simulink library "library_BCM"  (Simulink 8.2)
settings: Solver=ode45  StartTime=0.0  StopTime=10.0  RelTol=1e-3
undefined symbols (not defined in the file or in its folder): MPU_FOUR_CST, MPU_ONE_CST, MPU_THREE_CST, MPU_TWO_CST, MPU_ZERO_CST, NAMEOFTHEMODEL_SAMPLE_TIME_CST, slcm, TYP_MPU_REQUEST, TYP_MPU_REQUEST_2, TYP_MPU_STATUS, TYP_MPU_STATUS_2
libraries: Renault_Library x50, simulink x8, library_BCM x7
(part 1 of 3)
Description:
  | Library_BCM v1.0 :
  | Creation
  | Library_BCM v1.2 :
  | Corrections in Fault Manager
  | Library_BCM v1.3 :
  | Add MPU example in Modeling
  | Library_BCM v1.4 :
  | Add Block Conv_BoolToEvent_RisingEdge in Modeling
  | Library_BCM v1.5 :
  | Corrections in Fault Manager
  | Library_BCM v1.6 :
  | Add block EEPROM_SIMU in Validation
  | Library_BCM v.1.7 :
  | Add block EEPROM RNTBCI in Validation
  | Library_BCM v.1.8 :
  | Corrections of block EEPROM_SNAPSHOT in Fault Manager
  | Library_BCM v.1.9 :
  | Corrections of block EEPROM_SNAPSHOT in Fault Manager
  | Library_BCM v.1.10 :
  | Corrections of block CAN_FRAME_PRESENCE
  | Library_BCM v.1.11 :
  | Corrections of block EEPROM_SNAPSHOT in Fault Manager
  | Library_BCM v.1.12 :
  | Add  block PRESOAK_CHARGE_5CAL_7DAY
  | Library_BCM v.1.13 :
  | Optimisation of blocks in Fault Manager
  | Library_BCM v.1.14 :
  | correction of block EEPROM in Fault Manager
  | Library_BCM v.1.15 :
  | correction of block EEPROM in Fault Manager
  | Library_BCM v.1.16 :
  | correction of block EEPROM in Fault Manager
  | Library_BCM v.1.17 :
  | correction of block DTC & EEPROM in Fault Manager
  | Library_BCM v.1.18 :
  | correction of block EEPROM in Fault Manager
  | Library_BCM v.1.19 :
  | correction of block EEPROM in Fault Manager
  | Library_BCM v.1.20 :
  | correction of block DTC in Fault Manager
  | Library_BCM v.1.21 :
  | correction of block DTC in Fault Manager
  | Library_BCM v.1.22 :
  | correction of block INITIAL_PARAMETER in MIL Full Matlab
  | Library_BCM v.1.23 :
  | correction of block EEPROM in Fault Manager (RESET/RAZ)
  | Library_BCM v.1.24 :
  | add block RSA_Dynamic2DLockupTable : ver : 01.00 for clim waiting included in library lite
  | Library_BCM v.1.25 :
  | correction of block EEPROM in Fault Manager (constant type, QA FNR)
  | Library_BCM v.1.26 :
  | Correction of block RSA_Dynamic2DLockupTable to delete double inside
settings Model: Creator=p072376  LastModifiedBy=a003809

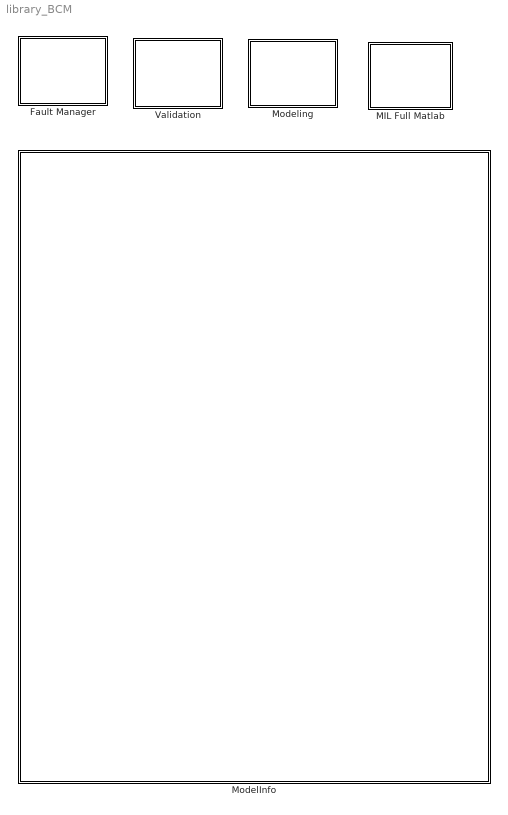
== system library_BCM ==
  Fault Manager : Subsystem
  MIL Full Matlab : Subsystem
  ModelInfo : Subsystem  LoadFcn=slcm LoadBlock;  InitFcn=slcm('UpdateAllCMBlocksInThisModelInit')  mask(CMBlock){InitialSaveTempField=, InitialBlockCM=None, BlockCM=None, Frame=on, SaveTempField=, DisplayStringWithTags=|, MaskDisplayString=library_BCM\nLibrary_BCM v1.0 : \nCreation\nLibrary_BCM v1.2 :\nCorrections in Fault Manager\nLibrary_BCM v1.3 :\nAdd MPU example in Modeling\nLibrary_BCM v1.4 :\nAdd Block Conv_BoolToEvent_RisingEdge in Modeling\nLibrary_BCM v1.5 :\nCorrections in Fault Manager\nLibrary_BCM v1.6 :\nAdd block EEPROM_SIMU in Validation\nLibrary_BCM v.1.7 :\nAdd block EEPROM RNTBCI in Validation\nLibrary_BCM v.1.8 :\nCorrections of block EEPROM_SNAPSHOT in Fault Manager\nLibrary_BCM v.1.9 :\nCorrections of block EEPROM_SNAPSHOT in Fault Manager\nLibrary_BCM v.1.10 :\nCorrections of block CAN_FRAME_PRESENCE\nLibrary_BCM v.1.11 :\nCorrections of block EEPROM_SNAPSHOT in Fault Manager\nLibrary_BCM v.1.12 :\nAdd  block PRESOAK_CHARGE_5CAL_7DAY\nLibrary_BCM v.1.13 :\nOptimisation of blocks in Fault Manager\nLibrary_BCM v.1.14 :\ncorrection of block EEPROM in Fault Manager\nLibrary_BCM v.1.15 :\ncorrection of block EEPROM in Fault Manager\nLibrary_BCM v.1.16 :\ncorrection of block EEPROM in Fault Manager\nLibrary_BCM v.1.17 :\ncorrection of block DTC & EEPROM in Fault Manager\nLibrary_BCM v.1.18 :\ncorrection of block EEPROM in Fault Manager\nLibrary_BCM v.1.19 :\ncorrection of block EEPROM in Fault Manager\nLibrary_BCM v.1.20 :\ncorrection of block DTC in Fault Manager\nLibrary_BCM v.1.21 :\ncorrection of block DTC in Fault Manager\nLibrary_BCM v.1.22 :\ncorrection of block INITIAL_PARAMETER in MIL Full Matlab\nLibrary_BCM v.1.23 :\ncorrection of block EEPROM in Fault Manager (RESET/RAZ)\nLibrary_BCM v.1.24 :\nadd block RSA_Dynamic2DLockupTable : ver : 01.00 for clim waiting included in library lite\nLibrary_BCM v.1.25 :\ncorrection of block EEPROM in Fault Manager (constant type, QA FNR)\nLibrary_BCM v.1.26 :\nCorrection of block RSA_Dynamic2DLockupTable to delete double inside, HorizontalTextAlignment=Center, LeftAlignmentValue=0.5, SourceBlockDiagram=library_BCM, TagMaxNumber=20, CMTag1=, CMTag2=, CMTag3=, CMTag4=, CMTag5=, CMTag6=, CMTag7=, CMTag8=, CMTag9=, CMTag10=, CMTag11=, CMTag12=, CMTag13=, CMTag14=, CMTag15=, CMTag16=, CMTag17=, CMTag18=, CMTag19=, CMTag20=}
      mask DisplayStringWithTags=|
      | %<ModelName>
      | %<Description>
      mask help: This block allows revision control information to be displayed within the model.
      settings: CopyFcn=slcm CopyBlock;  DeleteFcn=slcm Cancel;  PostSaveFcn=slcm('UpdateAllCMBlocksInThisModel')  NameChangeFcn=slcm Rename;  OpenFcn=slcm
      mask Display: text(str2num(LeftAlignmentValue), 0.5, MaskDisplayString, 'HorizontalAlignment', HorizontalTextAlignment)
  Modeling : Subsystem
  Validation : Subsystem

== system library_BCM/Fault Manager ==
  DTC : Subsystem  Tag=[RUNNABLE]  Description=|  mask{DTC_IDENTITY=928514, DTC_SNAPSHOT_NUMBER_CONV_CST=3, NUMBER_DTC_RECORD_IN_E2P_CST=2}
      | RQT_Fault_Manager_BCM_1_1
      | RQT_Fault_Manager_BCM_1_2
      | RQT_Fault_Manager_BCM_2_1
      | RQT_Fault_Manager_BCM_2_5
      mask prompts: DTC_IDENTITY "identification number DTC"; DTC_SNAPSHOT_NUMBER_CONV_CST "snapshot number"; NUMBER_DTC_RECORD_IN_E2P_CST "Number of DTC save in EEPROM"
  EEPROM_SNAPSHOT : Subsystem  mask{NUMBER_DTC_RECORD_IN_RAM_CST=178, NUMBER_DTC_RECORD_IN_E2P_CST=10, SNAPSHOT_NUMBER_CST=5, SNAPSHOT_MAX_LENGHT=32}
      mask prompts: NUMBER_DTC_RECORD_IN_RAM_CST "Number of DTC"; NUMBER_DTC_RECORD_IN_E2P_CST "Number of DTC save in EEPROM"; SNAPSHOT_NUMBER_CST "Number of snapshot"; SNAPSHOT_MAX_LENGHT "Snapshot max lenght (octet)"

== system library_BCM/MIL Full Matlab ==
  CAN_FRAME_PRESENCE : Subsystem  Tag=[REUSABLE]
  CONVERT_INT_TO_ENUM_WITH_UNAVAILABLE_VALUE : Subsystem  mask{UnavailableValue=3}
      mask prompts: UnavailableValue "Unavailable Value"
  COUNTER_INC : Subsystem
  INITIAL_PARAMETER : Subsystem  mask{INITIAL_VALUE=[9 99 100]}
  MONITORED_FRAME_MANAGEMENT : Subsystem  mask{CycleTime=10}
      mask prompts: CycleTime "Cycle Time in Ms"
  MUX_SEND_FRAME : Subsystem  mask(RSA_MuxSendFrame){FRAME_PERIOD=10, MAX_PARAMETER=3}
      mask prompts: FRAME_PERIOD "Period (ms)"; MAX_PARAMETER "Max counter"
      mask help:
      | Send a frame periodically or when an event parameter is updated.
      | - Period: Frame period (in ms)
      | Version : 01.00
      mask Help:
      | Send a frame periodically or when an event parameter is updated.
      | - Period: Frame period (in ms)
      | Version : 01.00
      mask Display:
      | disp('Mux Send Frame Simulink')
      | port_label('Input',1,'CAN_V_EMISSION_ON')
      | port_label('Input',2,'EVENT_DATA')
      | port_label('Output',1,'FRAME_SEND')
  NOT_MONITORED_FRAME_MANAGEMENT : Subsystem  mask{CycleTime=10}
      mask prompts: CycleTime "Cycle Time in Ms"
  Scheduler : Stateflow chart  TreatAsAtomicUnit=on
  Scheduling : Subsystem  TreatAsAtomicUnit=on  mask{Frequency=10}
  Scheduling0 : Subsystem  TreatAsAtomicUnit=on  mask{Frequency=10}
  TIME_OUT_EVENT_AT_INIT : Subsystem  mask{InitialConditions=true}
      mask prompts: InitialConditions "Initial Conditions"
      mask init:
      | %check_non_inherited_samp(Ts);
      | UDVAL = uint32(1e6);
      | INIVAL = uint32(0);
      | Ps=uint32(1);
      mask Display:
      | fprintf('tm(Event,dly)')
      | port_label('output', 1, 'Out')
      | port_label('input', 1, 'In')
      | port_label('input', 2, 'dly')

== system library_BCM/ModelInfo ==
  EmptySubsystem : Subsystem

== system library_BCM/Modeling ==
  Conv_BoolToEvent : Subsystem
      mask help: This block convert Boolean to a TYP_EVENT when the input change
  Conv_BoolToEvent_RisingEdge : Subsystem
      mask help: This block convert Boolean to a TYP_EVENT at the rising edge of input
  Conv_EventToBool : Subsystem
      mask help: This block convert TYP_EVENT to a boolean
  MPU_BOOLEAN_EXAMPLE : Subsystem
  MPU_ENUMERATED_EXAMPLE : Subsystem
  PRESOAK_CHARGE_5CAL_7DAY : Subsystem
      mask Display: disp('MODULO_Curenttime')
  RSA_Dynamic2DLookupTable_V01_00 : Subsystem  Tag=[LIB]  mask(RSA_Dynamic2DLookupTable){}
      mask help:
      | 2D Dynamic Lookup Table performs an interpolation of inputs based on dynamic breakpoints and Lookup Table values.
      | Inputs should be in the following format:
      | 1. x: Scalar x-coordinate
      | 2. y: Scalar y-coordinate
      | 3: x_breakpoints: Monotonically increasing vector of breakpoints for x-data
      | 4: y_breakpoints: Monotonically increasing vector of breakpoints for y-data
      | 5. table: Tabular data. Number of rows and columns in table should match the length of the breakpoints vector.
      |
      | Version : 01.00
      settings: AttributesFormatString=%<MaskType> : Ver : 01.00
      mask Help: eval(['open([','''\\F-khepri\shared\DIM-DCMAP-CGMP\66161\Shared_MatLab\Tools_DCMAP\Common_Library_MBDR\Library\Common_Library\Help\RLV_RSA_Dynamic2D_Spec_v01_00.pdf''','])'])
  TIME_OUT : Subsystem  mask{InitialConditions=false}
      mask prompts: InitialConditions "Parameters"
      mask init:
      | %check_non_inherited_samp(Ts);
      | UDVAL = uint32(1e6);
      | INIVAL = uint32(0);
      | Ps=uint32(1);
      mask DialogControl ParameterTabVar0 Prompt: Initial Conditions
      mask Display:
      | fprintf('tm(Event,dly)')
      | port_label('output', 1, 'Out')
      | port_label('input', 1, 'In')
      | port_label('input', 2, 'dly')
  Timer_Conversion : Subsystem  mask{NAMEOFTHEMODEL_SAMPLE_TIME_CST=NAMEOFTHEMODEL_SAMPLE_TIME_CST}
      mask prompts: NAMEOFTHEMODEL_SAMPLE_TIME_CST "Name of the sample time constant define in the constant file .m of the model"
      mask help: Timer Conversion for BCM/HFM
      mask init:
      | ZERO_CST = 0;

== system library_BCM/Validation ==
  EEPROM : Subsystem  mask(EEPROM simulation with ECU Reset){}
      mask help: Manage EEPROM for jFTL Simulation with ECU_RESET
  EEPROM_OLD : Subsystem  mask(EEPROM Simulation){}
      mask help: Manage EEPROM for jFTL Simulation
  EEPROM_SIMU : Subsystem  mask(EEPROM simulation with ECU Reset){}
      mask help: Manage EEPROM for jFTL Simulation with ECU_RESET

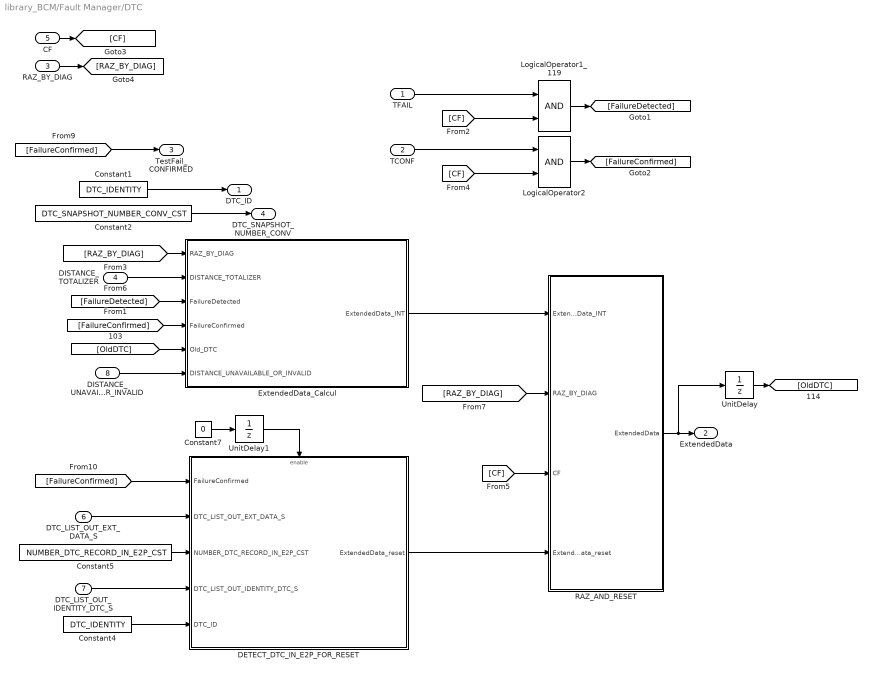
== system library_BCM/Fault Manager/DTC ==
  TFAIL : Inport  OutDataTypeStr=boolean
  TCONF : Inport  Port=2  OutDataTypeStr=boolean
  RAZ_BY_DIAG : Inport  Port=3  OutDataTypeStr=boolean
  DISTANCE_TOTALIZER : Inport  Port=4  OutDataTypeStr=uint32
      settings: CopyFcn=if exist('tl_check_ports','file'), tl_check_ports(gcbh); end  NameChangeFcn=if exist('tl_check_ports','file'), tl_check_ports(gcbh); end
  CF : Inport  Port=5  OutDataTypeStr=boolean
  DTC_LIST_OUT_EXT_DATA_S : Inport  Port=6  OutDataTypeStr=uint32  PortDimensions=NUMBER_DTC_RECORD_IN_E2P_CST
      settings: AttributesFormatString=Type : %<OutDataTypeStr>
  DTC_LIST_OUT_IDENTITY_DTC_S : Inport  Port=7  OutDataTypeStr=uint32  PortDimensions=NUMBER_DTC_RECORD_IN_E2P_CST
      settings: AttributesFormatString=Type : %<OutDataTypeStr>
  DISTANCE_UNAVAILABLE_OR_INVALID : Inport  Port=8  OutDataTypeStr=boolean
  Constant1 : Constant  Value=DTC_IDENTITY  OutDataTypeStr=Inherit: Inherit via back propagation  SampleTime=-1
  Constant2 : Constant  Value=DTC_SNAPSHOT_NUMBER_CONV_CST  OutDataTypeStr=Inherit: Inherit via back propagation  SampleTime=-1
  Constant4 : Constant  Value=DTC_IDENTITY  OutDataTypeStr=uint32  SampleTime=-1
  Constant5 : Constant  Value=NUMBER_DTC_RECORD_IN_E2P_CST  OutDataTypeStr=uint32  SampleTime=-1
  Constant7 : Constant  Value=0  OutDataTypeStr=boolean  SampleTime=-1
  DETECT_DTC_IN_E2P_FOR_RESET : Subsystem  Description=|  TreatAsAtomicUnit=on
      | RQT_Fault_Manager_BCM_2_2  
      | RQT_Fault_Manager_BCM_4_1  
      | RQT_Fault_Manager_BCM_4_2_a
  ExtendedData_Calcul : Subsystem  Description=|
      | RQT_Fault_Manager_BCM_2_3
      | RQT_Fault_Manager_BCM_2_4
  LogicalOperator1_119 : Logic  Tag=struct('inputs','2','comment',struct('text','','placement',1),'logdata',struct('maxnumvals',inf,'plotchannels',[],'loggingmode',3,'channels',1),'operator','AND','output',struct('variable','','description','','name','$S_$B','address','','class','default','type','Bool','unit',''),'scalingvalid',0,'date',730486)  OutDataTypeStr=boolean
  LogicalOperator2 : Logic  Tag=struct('inputs','2','comment',struct('text','','placement',1),'logdata',struct('maxnumvals',inf,'plotchannels',[],'loggingmode',3,'channels',1),'operator','AND','output',struct('variable','','description','','name','$S_$B','address','','class','default','type','Bool','unit',''),'scalingvalid',0,'date',730486)  OutDataTypeStr=boolean
  RAZ_AND_RESET : Subsystem  Description=|
      | RQT_Fault_Manager_BCM_1_6
      | RQT_Fault_Manager_BCM_1_7
      | RQT_Fault_Manager_BCM_2_8
  UnitDelay : UnitDelay  SampleTime=-1
      settings: AttributesFormatString=IC = %<X0>
  UnitDelay1 : UnitDelay  InitialCondition=1  SampleTime=-1
      settings: AttributesFormatString=IC = %<X0>
  DTC_ID : Outport  OutDataTypeStr=uint32  InitialOutput=0
      settings: CopyFcn=if exist('tl_check_ports','file'), tl_check_ports(gcbh); end  NameChangeFcn=if exist('tl_check_ports','file'), tl_check_ports(gcbh); end
  ExtendedData : Outport  Port=2  OutDataTypeStr=uint32  InitialOutput=0
      settings: CopyFcn=if exist('tl_check_ports','file'), tl_check_ports(gcbh); end  NameChangeFcn=if exist('tl_check_ports','file'), tl_check_ports(gcbh); end
  TestFail_CONFIRMED : Outport  Port=3  OutDataTypeStr=boolean  InitialOutput=0
      settings: CopyFcn=if exist('tl_check_ports','file'), tl_check_ports(gcbh); end  NameChangeFcn=if exist('tl_check_ports','file'), tl_check_ports(gcbh); end
  DTC_SNAPSHOT_NUMBER_CONV : Outport  Port=4  OutDataTypeStr=uint8  InitialOutput=0
      settings: CopyFcn=if exist('tl_check_ports','file'), tl_check_ports(gcbh); end  NameChangeFcn=if exist('tl_check_ports','file'), tl_check_ports(gcbh); end
  wires:
  [CF] -> LogicalOperator2/2
  [CF] -> LogicalOperator1_119/2
  RAZ_BY_DIAG/1 -> [RAZ_BY_DIAG]
  [OldDTC] -> ExtendedData_Calcul/5(Old_DTC)
  [RAZ_BY_DIAG] -> RAZ_AND_RESET/2(RAZ_BY_DIAG)
  DETECT_DTC_IN_E2P_FOR_RESET/1(ExtendedData_reset) -> RAZ_AND_RESET/4(ExtendedData_reset)
  ExtendedData_Calcul/1(ExtendedData_INT) -> RAZ_AND_RESET/1(ExtendedData_INT)
  [FailureConfirmed] -> ExtendedData_Calcul/4(FailureConfirmed)
  [FailureDetected] -> ExtendedData_Calcul/3(FailureDetected)
  RAZ_AND_RESET/1(ExtendedData) -> UnitDelay/1, ExtendedData/1
  UnitDelay/1 -> [OldDTC]
  DISTANCE_TOTALIZER/1 -> ExtendedData_Calcul/2(DISTANCE_TOTALIZER)
  [RAZ_BY_DIAG] -> ExtendedData_Calcul/1(RAZ_BY_DIAG)
  UnitDelay1/1 -> DETECT_DTC_IN_E2P_FOR_RESET/Enable
  Constant7/1 -> UnitDelay1/1
  Constant4/1 -> DETECT_DTC_IN_E2P_FOR_RESET/5(DTC_ID)
  DTC_LIST_OUT_IDENTITY_DTC_S/1 -> DETECT_DTC_IN_E2P_FOR_RESET/4(DTC_LIST_OUT_IDENTITY_DTC_S)
  Constant5/1 -> DETECT_DTC_IN_E2P_FOR_RESET/3(NUMBER_DTC_RECORD_IN_E2P_CST)
  DTC_LIST_OUT_EXT_DATA_S/1 -> DETECT_DTC_IN_E2P_FOR_RESET/2(DTC_LIST_OUT_EXT_DATA_S)
  [FailureConfirmed] -> DETECT_DTC_IN_E2P_FOR_RESET/1(FailureConfirmed)
  Constant2/1 -> DTC_SNAPSHOT_NUMBER_CONV/1
  Constant1/1 -> DTC_ID/1
  [FailureConfirmed] -> TestFail_CONFIRMED/1
  TCONF/1 -> LogicalOperator2/1
  LogicalOperator2/1 -> [FailureConfirmed]
  LogicalOperator1_119/1 -> [FailureDetected]
  TFAIL/1 -> LogicalOperator1_119/1
  CF/1 -> [CF]
  [CF] -> RAZ_AND_RESET/3(CF)
  DISTANCE_UNAVAILABLE_OR_INVALID/1 -> ExtendedData_Calcul/6(DISTANCE_UNAVAILABLE_OR_INVALID)

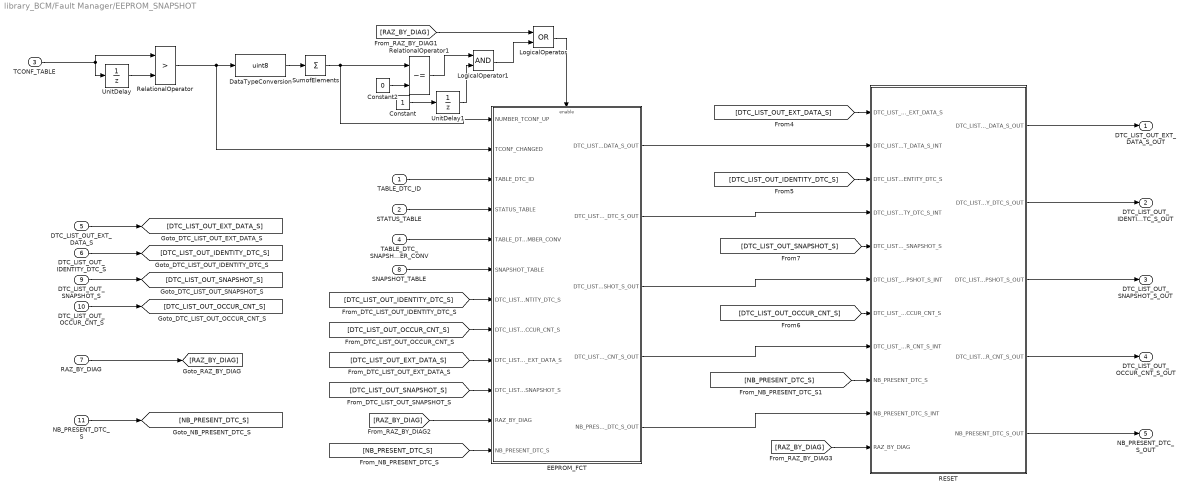
== system library_BCM/Fault Manager/EEPROM_SNAPSHOT ==
  TABLE_DTC_ID : Inport  OutDataTypeStr=uint32
      settings: AttributesFormatString=Type : %<OutDataTypeStr>
  STATUS_TABLE : Inport  Port=2  OutDataTypeStr=uint32  PortDimensions=NUMBER_DTC_RECORD_IN_RAM_CST
      settings: AttributesFormatString=Type : %<OutDataTypeStr>
  TCONF_TABLE : Inport  Port=3  OutDataTypeStr=boolean  PortDimensions=NUMBER_DTC_RECORD_IN_RAM_CST
      settings: AttributesFormatString=Type : %<OutDataTypeStr>
  TABLE_DTC_SNAPSHOT_NUMBER_CONV : Inport  Port=4  OutDataTypeStr=uint8  PortDimensions=NUMBER_DTC_RECORD_IN_RAM_CST
      settings: AttributesFormatString=Type : %<OutDataTypeStr>
  DTC_LIST_OUT_EXT_DATA_S : Inport  Port=5  OutDataTypeStr=uint32  PortDimensions=NUMBER_DTC_RECORD_IN_E2P_CST
      settings: AttributesFormatString=Type : %<OutDataTypeStr>
  DTC_LIST_OUT_IDENTITY_DTC_S : Inport  Port=6  OutDataTypeStr=uint32  PortDimensions=NUMBER_DTC_RECORD_IN_E2P_CST
      settings: AttributesFormatString=Type : %<OutDataTypeStr>
  RAZ_BY_DIAG : Inport  Port=7  OutDataTypeStr=boolean
      settings: AttributesFormatString=Type : %<OutDataTypeStr>
  SNAPSHOT_TABLE : Inport  Port=8  OutDataTypeStr=uint8  PortDimensions=[SNAPSHOT_MAX_LENGHT SNAPSHOT_NUMBER_CST]
      settings: AttributesFormatString=Type : %<OutDataTypeStr>
  DTC_LIST_OUT_SNAPSHOT_S : Inport  Port=9  OutDataTypeStr=uint8  PortDimensions=[SNAPSHOT_MAX_LENGHT NUMBER_DTC_RECORD_IN_E2P_CST]
      settings: AttributesFormatString=Type : %<OutDataTypeStr>
  DTC_LIST_OUT_OCCUR_CNT_S : Inport  Port=10  OutDataTypeStr=uint8  PortDimensions=NUMBER_DTC_RECORD_IN_E2P_CST
      settings: AttributesFormatString=Type : %<OutDataTypeStr>
  NB_PRESENT_DTC_S : Inport  Port=11  OutDataTypeStr=uint8
      settings: AttributesFormatString=Type : %<OutDataTypeStr>
  Constant : Constant  OutDataTypeStr=Inherit: Inherit via back propagation  SampleTime=-1
  Constant2 : Constant  Value=0  OutDataTypeStr=Inherit: Inherit via back propagation  SampleTime=-1
  DataTypeConversion : DataTypeConversion  OutDataTypeStr=uint8  RndMeth=Zero
      settings: AttributesFormatString=Saturation:%<SaturateOnIntegerOverflow>
  EEPROM_FCT : Subsystem
  LogicalOperator : Logic  Operator=OR  OutDataTypeStr=boolean
  LogicalOperator1 : Logic  OutDataTypeStr=boolean
  RESET : Subsystem  Description=RQT_Fault_Manager_BCM_4_2_a
  RelationalOperator : RelationalOperator  Operator=>  OutDataTypeStr=boolean  InputSameDT=on
  RelationalOperator1 : RelationalOperator  Operator=~=  OutDataTypeStr=boolean  InputSameDT=on
  SumofElements : Sum  Inputs=+  OutDataTypeStr=Inherit: Inherit via back propagation  RndMeth=Zero  InputSameDT=on
  UnitDelay : UnitDelay  SampleTime=-1
      settings: AttributesFormatString=IC = %<X0>
  UnitDelay1 : UnitDelay  SampleTime=-1
      settings: AttributesFormatString=IC = %<X0>
  DTC_LIST_OUT_EXT_DATA_S_OUT : Outport  OutDataTypeStr=uint32  PortDimensions=NUMBER_DTC_RECORD_IN_E2P_CST
      settings: AttributesFormatString=Type : %<OutDataTypeStr>\nInit :%<InitialOutput>
  DTC_LIST_OUT_IDENTITY_DTC_S_OUT : Outport  Port=2  OutDataTypeStr=uint32  PortDimensions=NUMBER_DTC_RECORD_IN_E2P_CST
      settings: AttributesFormatString=Type : %<OutDataTypeStr>\nInit :%<InitialOutput>
  DTC_LIST_OUT_SNAPSHOT_S_OUT : Outport  Port=3  OutDataTypeStr=uint8  PortDimensions=[SNAPSHOT_MAX_LENGHT NUMBER_DTC_RECORD_IN_E2P_CST]
      settings: AttributesFormatString=Type : %<OutDataTypeStr>\nInit :%<InitialOutput>
  DTC_LIST_OUT_OCCUR_CNT_S_OUT : Outport  Port=4  OutDataTypeStr=uint8  PortDimensions=NUMBER_DTC_RECORD_IN_E2P_CST
      settings: AttributesFormatString=Type : %<OutDataTypeStr>\nInit :%<InitialOutput>
  NB_PRESENT_DTC_S_OUT : Outport  Port=5  OutDataTypeStr=uint8
      settings: AttributesFormatString=Type : %<OutDataTypeStr>\nInit :%<InitialOutput>
  wires:
  [DTC_LIST_OUT_OCCUR_CNT_S] -> RESET/7(DTC_LIST_OUT_OCCUR_CNT_S)
  [DTC_LIST_OUT_SNAPSHOT_S] -> RESET/5(DTC_LIST_OUT_SNAPSHOT_S)
  [DTC_LIST_OUT_IDENTITY_DTC_S] -> RESET/3(DTC_LIST_OUT_IDENTITY_DTC_S)
  [DTC_LIST_OUT_EXT_DATA_S] -> RESET/1(DTC_LIST_OUT_EXT_DATA_S)
  RESET/4(DTC_LIST_OUT_OCCUR_CNT_S_OUT) -> DTC_LIST_OUT_OCCUR_CNT_S_OUT/1
  RESET/3(DTC_LIST_OUT_SNAPSHOT_S_OUT) -> DTC_LIST_OUT_SNAPSHOT_S_OUT/1
  RESET/2(DTC_LIST_OUT_IDENTITY_DTC_S_OUT) -> DTC_LIST_OUT_IDENTITY_DTC_S_OUT/1
  RESET/1(DTC_LIST_OUT_EXT_DATA_S_OUT) -> DTC_LIST_OUT_EXT_DATA_S_OUT/1
  DTC_LIST_OUT_OCCUR_CNT_S/1 -> [DTC_LIST_OUT_OCCUR_CNT_S]
  DTC_LIST_OUT_SNAPSHOT_S/1 -> [DTC_LIST_OUT_SNAPSHOT_S]
  DTC_LIST_OUT_IDENTITY_DTC_S/1 -> [DTC_LIST_OUT_IDENTITY_DTC_S]
  DTC_LIST_OUT_EXT_DATA_S/1 -> [DTC_LIST_OUT_EXT_DATA_S]
  TABLE_DTC_ID/1 -> EEPROM_FCT/3(TABLE_DTC_ID)
  STATUS_TABLE/1 -> EEPROM_FCT/4(STATUS_TABLE)
  TABLE_DTC_SNAPSHOT_NUMBER_CONV/1 -> EEPROM_FCT/5(TABLE_DTC_SNAPSHOT_NUMBER_CONV)
  SNAPSHOT_TABLE/1 -> EEPROM_FCT/6(SNAPSHOT_TABLE)
  EEPROM_FCT/1(DTC_LIST_OUT_EXT_DATA_S_OUT) -> RESET/2(DTC_LIST_OUT_EXT_DATA_S_INT)
  EEPROM_FCT/2(DTC_LIST_OUT_IDENTITY_DTC_S_OUT) -> RESET/4(DTC_LIST_OUT_IDENTITY_DTC_S_INT)
  EEPROM_FCT/3(DTC_LIST_OUT_SNAPSHOT_S_OUT) -> RESET/6(DTC_LIST_OUT_SNAPSHOT_S_INT)
  EEPROM_FCT/4(DTC_LIST_OUT_OCCUR_CNT_S_OUT) -> RESET/8(DTC_LIST_OUT_OCCUR_CNT_S_INT)
  TCONF_TABLE/1 -> RelationalOperator/1, UnitDelay/1
  UnitDelay/1 -> RelationalOperator/2
  RelationalOperator/1 -> EEPROM_FCT/2(TCONF_CHANGED), DataTypeConversion/1
  DataTypeConversion/1 -> SumofElements/1
  SumofElements/1 -> RelationalOperator1/1, EEPROM_FCT/1(NUMBER_TCONF_UP)
  Constant2/1 -> RelationalOperator1/2
  [DTC_LIST_OUT_IDENTITY_DTC_S] -> EEPROM_FCT/7(DTC_LIST_OUT_IDENTITY_DTC_S)
  [DTC_LIST_OUT_OCCUR_CNT_S] -> EEPROM_FCT/8(DTC_LIST_OUT_OCCUR_CNT_S)
  [DTC_LIST_OUT_SNAPSHOT_S] -> EEPROM_FCT/10(DTC_LIST_OUT_SNAPSHOT_S)
  [DTC_LIST_OUT_EXT_DATA_S] -> EEPROM_FCT/9(DTC_LIST_OUT_EXT_DATA_S)
  RAZ_BY_DIAG/1 -> [RAZ_BY_DIAG]
  [RAZ_BY_DIAG] -> LogicalOperator/1
  LogicalOperator/1 -> EEPROM_FCT/Enable
  [RAZ_BY_DIAG] -> EEPROM_FCT/11(RAZ_BY_DIAG)
  Constant/1 -> UnitDelay1/1
  RelationalOperator1/1 -> LogicalOperator1/1
  LogicalOperator1/1 -> LogicalOperator/2
  UnitDelay1/1 -> LogicalOperator1/2
  EEPROM_FCT/5(NB_PRESENT_DTC_S_OUT) -> RESET/10(NB_PRESENT_DTC_S_INT)
  NB_PRESENT_DTC_S/1 -> [NB_PRESENT_DTC_S]
  [NB_PRESENT_DTC_S] -> EEPROM_FCT/12(NB_PRESENT_DTC_S)
  [NB_PRESENT_DTC_S] -> RESET/9(NB_PRESENT_DTC_S)
  RESET/5(NB_PRESENT_DTC_S_OUT) -> NB_PRESENT_DTC_S_OUT/1
  [RAZ_BY_DIAG] -> RESET/11(RAZ_BY_DIAG)

== system library_BCM/MIL Full Matlab/CAN_FRAME_PRESENCE ==
  NETWORK_OPERATES : Inport
      settings: AttributesFormatString=Type : %<OutDataTypeStr>
  XXX_FRAME_ABSENT : Inport  Port=2
      settings: AttributesFormatString=Type : %<OutDataTypeStr>
  XXX_FRAME_RECEIVED : Inport  Port=3
      settings: AttributesFormatString=Type : %<OutDataTypeStr>
  DataTypeConversion : DataTypeConversion  OutDataTypeStr=boolean  RndMeth=Zero
      settings: AttributesFormatString=Saturation:%<SaturateOnIntegerOverflow>
  DataTypeConversion1 : DataTypeConversion  OutDataTypeStr=boolean  RndMeth=Zero
      settings: AttributesFormatString=Saturation:%<SaturateOnIntegerOverflow>
  LogicalOperator : Logic  Operator=NOT  OutDataTypeStr=boolean
  LogicalOperator1 : Logic  Operator=OR  OutDataTypeStr=boolean
  LogicalOperator4 : Logic  Operator=NOT  OutDataTypeStr=boolean
  RSA_DetectIncrease : Renault_Library/Complex blocks/Logic & Bit Operations/RSA_DetectIncrease  Tag=[LIB]  vinit=false
      settings: AttributesFormatString=%<MaskType> : Ver : 01.02\nInitial condition: %<vinit>
  RSA_DetectIncrease1 : Renault_Library/Complex blocks/Logic & Bit Operations/RSA_DetectIncrease  Tag=[LIB]  vinit=false
      settings: AttributesFormatString=%<MaskType> : Ver : 01.02\nInitial condition: %<vinit>
  RSA_SRFlipFlopSetPrioritary : Renault_Library/Complex blocks/Flip-Flop/RSA_SRFlipFlopSetPrioritary  Tag=[LIB]  init=true
      settings: AttributesFormatString=%<MaskType> : Ver : 01.02\n<init=%<init>>
  CAN_XXX_PRESENT : Outport
      settings: AttributesFormatString=Type : %<OutDataTypeStr>
  wires:
  XXX_FRAME_RECEIVED/1 -> DataTypeConversion/1
  XXX_FRAME_ABSENT/1 -> DataTypeConversion1/1
  DataTypeConversion/1 -> RSA_DetectIncrease/1
  DataTypeConversion1/1 -> RSA_DetectIncrease1/1
  LogicalOperator1/1 -> RSA_SRFlipFlopSetPrioritary/1
  NETWORK_OPERATES/1 -> LogicalOperator/1
  LogicalOperator/1 -> LogicalOperator1/1
  RSA_DetectIncrease/1 -> RSA_SRFlipFlopSetPrioritary/2
  RSA_SRFlipFlopSetPrioritary/1 -> LogicalOperator4/1
  RSA_DetectIncrease1/1 -> LogicalOperator1/2
  LogicalOperator4/1 -> CAN_XXX_PRESENT/1

== system library_BCM/MIL Full Matlab/CONVERT_INT_TO_ENUM_WITH_UNAVAILABLE_VALUE ==
  XI_DATA : Inport
      settings: AttributesFormatString=Type : %<OutDataTypeStr>
  FAME_INC : Inport  Port=2  OutDataTypeStr=uint8
      settings: AttributesFormatString=Type : %<OutDataTypeStr>
  BlockConvert2 : DataTypeConversion  RndMeth=Zero
  BlockConvert3 : DataTypeConversion  RndMeth=Zero
  Constant3 : Constant  Value=UnavailableValue  OutDataTypeStr=uint32
  Constant4 : Constant  Value=3  OutDataTypeStr=uint8
  RelationalOperator : RelationalOperator  Operator=~=  OutDataTypeStr=boolean
  Switch : Switch  RndMeth=Zero
  DATA : Outport
      settings: AttributesFormatString=Type : %<OutDataTypeStr>\nInit :%<InitialOutput>
  wires:
  Constant3/1 -> BlockConvert3/1
  Constant4/1 -> RelationalOperator/2
  Switch/1 -> BlockConvert2/1
  RelationalOperator/1 -> Switch/2
  XI_DATA/1 -> Switch/1
  FAME_INC/1 -> RelationalOperator/1
  BlockConvert2/1 -> DATA/1
  BlockConvert3/1 -> Switch/3

== system library_BCM/MIL Full Matlab/COUNTER_INC ==
  EVENT : Inport
  Add : Sum  RndMeth=Zero
  Constant6 : Constant  OutDataTypeStr=uint8
  Switch3 : Switch  Criteria=u2 ~= 0  RndMeth=Zero  InputSameDT=on
      settings: AttributesFormatString=Criteria=%<Criteria>
  UnitDelay2 : UnitDelay  InitialCondition=false  SampleTime=-1
      settings: AttributesFormatString=IC = %<X0>
  COUNTER : Outport
      settings: AttributesFormatString=Init :%<InitialOutput>
  wires:
  [FRAME_INC] -> Add/1
  [FRAME_INC] -> Switch3/3
  UnitDelay2/1 -> [FRAME_INC]
  Switch3/1 -> UnitDelay2/1, COUNTER/1
  Add/1 -> Switch3/1
  Constant6/1 -> Add/2
  EVENT/1 -> Switch3/2

== system library_BCM/MIL Full Matlab/INITIAL_PARAMETER ==
  PAR_I_TM_TP : Inport
  Constant8 : Constant  Value=false  OutDataTypeStr=uint32
  Constant9 : Constant  Value=INITIAL_VALUE  OutDataTypeStr=Inherit: Inherit via back propagation
  DataTypeConversion1 : DataTypeConversion  OutDataTypeStr=uint32
  DataTypeConversion2 : DataTypeConversion
  DataTypeConversion3 : DataTypeConversion
  LogicalOperator : Logic  Operator=NOT  OutDataTypeStr=boolean
  RSA_DetectChange : Renault_Library/Complex blocks/Logic & Bit Operations/RSA_DetectChange  Tag=[LIB]  vinit=false
      settings: AttributesFormatString=%<MaskType> : Ver : 01.02\nInitial condition: %<vinit>
  RSA_DetectChange1 : Renault_Library/Complex blocks/Logic & Bit Operations/RSA_DetectChange  Tag=[LIB]  vinit=true
      settings: AttributesFormatString=%<MaskType> : Ver : 01.02\nInitial condition: %<vinit>
  RSA_SRFlipFlopSetPrioritary : Renault_Library/Complex blocks/Flip-Flop/RSA_SRFlipFlopSetPrioritary  Tag=[LIB]  init=false
      settings: AttributesFormatString=%<MaskType> : Ver : 01.02\n<init=%<init>>
  Switch : Switch  Criteria=u2 ~= 0
  TM_TP : Outport
  wires:
  Constant8/1 -> RSA_DetectChange1/1
  RSA_SRFlipFlopSetPrioritary/1 -> LogicalOperator/1
  PAR_I_TM_TP/1 -> DataTypeConversion2/1, Switch/1
  Switch/1 -> TM_TP/1
  Constant9/1 -> DataTypeConversion1/1
  LogicalOperator/1 -> Switch/2
  RSA_DetectChange1/1 -> RSA_SRFlipFlopSetPrioritary/1
  RSA_DetectChange/1 -> RSA_SRFlipFlopSetPrioritary/2
  DataTypeConversion2/1 -> RSA_DetectChange/1
  DataTypeConversion1/1 -> DataTypeConversion3/1
  DataTypeConversion3/1 -> Switch/3

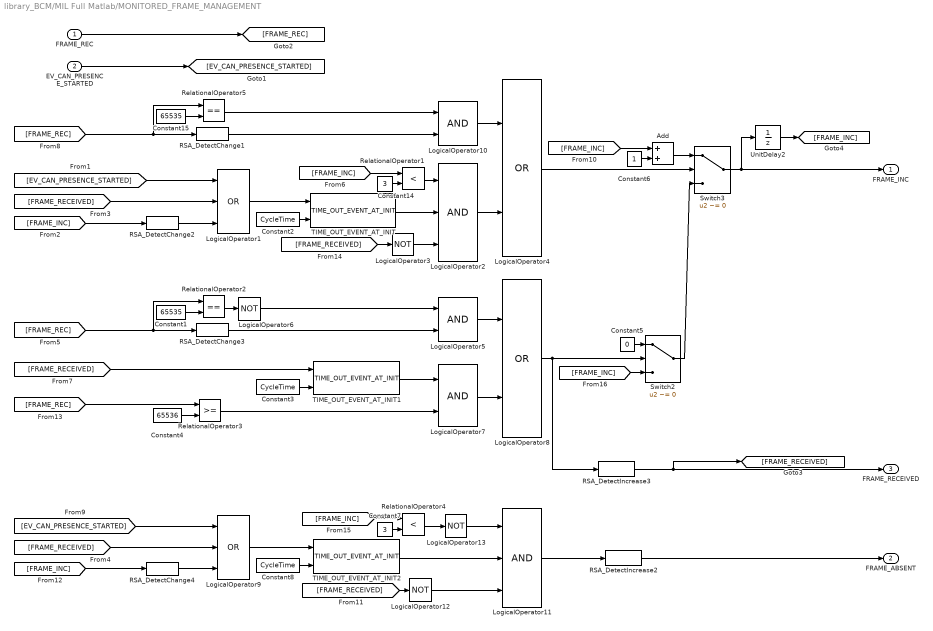
== system library_BCM/MIL Full Matlab/MONITORED_FRAME_MANAGEMENT ==
  FRAME_REC : Inport  OutDataTypeStr=uint32
      settings: AttributesFormatString=Type : %<OutDataTypeStr>
  EV_CAN_PRESENCE_STARTED : Inport  Port=2  OutDataTypeStr=boolean
      settings: AttributesFormatString=Type : %<OutDataTypeStr>
  Add : Sum  RndMeth=Zero
  Constant1 : Constant  Value=65535  OutDataTypeStr=uint32
  Constant14 : Constant  Value=3  OutDataTypeStr=uint8
  Constant15 : Constant  Value=65535  OutDataTypeStr=uint32
  Constant2 : Constant  Value=CycleTime  OutDataTypeStr=Inherit: Inherit via back propagation
  Constant3 : Constant  Value=CycleTime  OutDataTypeStr=Inherit: Inherit via back propagation
  Constant4 : Constant  Value=65536  OutDataTypeStr=uint32
  Constant5 : Constant  Value=0  OutDataTypeStr=uint8
  Constant6 : Constant  OutDataTypeStr=uint8
  Constant7 : Constant  Value=3  OutDataTypeStr=uint8
  Constant8 : Constant  Value=CycleTime  OutDataTypeStr=Inherit: Inherit via back propagation
  LogicalOperator1 : Logic  Operator=OR  Inputs=3  OutDataTypeStr=boolean
  LogicalOperator10 : Logic  OutDataTypeStr=boolean
  LogicalOperator11 : Logic  Inputs=3  OutDataTypeStr=boolean
  LogicalOperator{3,6,12..13} (4 alike) : Logic  Operator=NOT  OutDataTypeStr=boolean
  LogicalOperator2 : Logic  Inputs=3  OutDataTypeStr=boolean
  LogicalOperator4 : Logic  Operator=OR  OutDataTypeStr=boolean
  LogicalOperator5 : Logic  OutDataTypeStr=boolean
  LogicalOperator7 : Logic  OutDataTypeStr=boolean
  LogicalOperator8 : Logic  Operator=OR  OutDataTypeStr=boolean
  LogicalOperator9 : Logic  Operator=OR  Inputs=3  OutDataTypeStr=boolean
  RSA_DetectChange1 : Renault_Library/Complex blocks/Logic & Bit Operations/RSA_DetectChange  Tag=[LIB]  vinit=65535
      settings: AttributesFormatString=%<MaskType> : Ver : 01.02\nInitial condition: %<vinit>
  RSA_DetectChange2 : Renault_Library/Complex blocks/Logic & Bit Operations/RSA_DetectChange  Tag=[LIB]  vinit=false
      settings: AttributesFormatString=%<MaskType> : Ver : 01.02\nInitial condition: %<vinit>
  RSA_DetectChange3 : Renault_Library/Complex blocks/Logic & Bit Operations/RSA_DetectChange  Tag=[LIB]  vinit=65535
      settings: AttributesFormatString=%<MaskType> : Ver : 01.02\nInitial condition: %<vinit>
  RSA_DetectChange4 : Renault_Library/Complex blocks/Logic & Bit Operations/RSA_DetectChange  Tag=[LIB]  vinit=false
      settings: AttributesFormatString=%<MaskType> : Ver : 01.02\nInitial condition: %<vinit>
  RSA_DetectIncrease2 : Renault_Library/Complex blocks/Logic & Bit Operations/RSA_DetectIncrease  Tag=[LIB]  vinit=false
      settings: AttributesFormatString=%<MaskType> : Ver : 01.02\nInitial condition: %<vinit>
  RSA_DetectIncrease3 : Renault_Library/Complex blocks/Logic & Bit Operations/RSA_DetectIncrease  Tag=[LIB]  vinit=false
      settings: AttributesFormatString=%<MaskType> : Ver : 01.02\nInitial condition: %<vinit>
  RelationalOperator1 : RelationalOperator  Operator=<  OutDataTypeStr=boolean  InputSameDT=on
  RelationalOperator2 : RelationalOperator  Operator===  OutDataTypeStr=boolean  InputSameDT=on
  RelationalOperator3 : RelationalOperator  OutDataTypeStr=boolean  InputSameDT=on
  RelationalOperator4 : RelationalOperator  Operator=<  OutDataTypeStr=boolean  InputSameDT=on
  RelationalOperator5 : RelationalOperator  Operator===  OutDataTypeStr=boolean  InputSameDT=on
  Switch2 : Switch  Criteria=u2 ~= 0  RndMeth=Zero  InputSameDT=on
      settings: AttributesFormatString=Criteria=%<Criteria>
  Switch3 : Switch  Criteria=u2 ~= 0  RndMeth=Zero  InputSameDT=on
      settings: AttributesFormatString=Criteria=%<Criteria>
  TIME_OUT_EVENT_AT_INIT : library_BCM/MIL Full Matlab/TIME_OUT_EVENT_AT_INIT  InitialConditions=false
  TIME_OUT_EVENT_AT_INIT1 : library_BCM/MIL Full Matlab/TIME_OUT_EVENT_AT_INIT  InitialConditions=false
  TIME_OUT_EVENT_AT_INIT2 : library_BCM/MIL Full Matlab/TIME_OUT_EVENT_AT_INIT  InitialConditions=false
  UnitDelay2 : UnitDelay  InitialCondition=false  SampleTime=-1
      settings: AttributesFormatString=IC = %<X0>
  FRAME_INC : Outport  OutDataTypeStr=uint8
      settings: AttributesFormatString=Type : %<OutDataTypeStr>\nInit :%<InitialOutput>
  FRAME_ABSENT : Outport  Port=2
      settings: AttributesFormatString=Type : %<OutDataTypeStr>\nInit :%<InitialOutput>
  FRAME_RECEIVED : Outport  Port=3
      settings: AttributesFormatString=Type : %<OutDataTypeStr>\nInit :%<InitialOutput>
  wires:
  [FRAME_INC] -> Switch2/3
  [FRAME_INC] -> Add/1
  UnitDelay2/1 -> [FRAME_INC]
  Switch3/1 -> UnitDelay2/1, FRAME_INC/1
  LogicalOperator13/1 -> LogicalOperator11/1
  Constant2/1 -> TIME_OUT_EVENT_AT_INIT/2
  Constant15/1 -> RelationalOperator5/2
  RelationalOperator5/1 -> LogicalOperator10/1
  RSA_DetectChange1/1 -> LogicalOperator10/2
  FRAME_REC/1 -> [FRAME_REC]
  [FRAME_REC] -> RelationalOperator5/1, RSA_DetectChange1/1
  EV_CAN_PRESENCE_STARTED/1 -> [EV_CAN_PRESENCE_STARTED]
  [FRAME_INC] -> RSA_DetectChange2/1
  [FRAME_RECEIVED] -> LogicalOperator1/2
  LogicalOperator1/1 -> TIME_OUT_EVENT_AT_INIT/1
  [FRAME_RECEIVED] -> LogicalOperator3/1
  LogicalOperator3/1 -> LogicalOperator2/3
  TIME_OUT_EVENT_AT_INIT/1 -> LogicalOperator2/2
  RelationalOperator1/1 -> LogicalOperator2/1
  [FRAME_INC] -> RelationalOperator1/1
  Constant14/1 -> RelationalOperator1/2
  LogicalOperator2/1 -> LogicalOperator4/2
  LogicalOperator10/1 -> LogicalOperator4/1
  Constant1/1 -> RelationalOperator2/2
  RelationalOperator2/1 -> LogicalOperator6/1
  RSA_DetectChange3/1 -> LogicalOperator5/2
  [FRAME_REC] -> RSA_DetectChange3/1, RelationalOperator2/1
  LogicalOperator6/1 -> LogicalOperator5/1
  [FRAME_RECEIVED] -> TIME_OUT_EVENT_AT_INIT1/1
  TIME_OUT_EVENT_AT_INIT1/1 -> LogicalOperator7/1
  Constant4/1 -> RelationalOperator3/2
  RelationalOperator3/1 -> LogicalOperator7/2
  [FRAME_REC] -> RelationalOperator3/1
  LogicalOperator5/1 -> LogicalOperator8/1
  LogicalOperator7/1 -> LogicalOperator8/2
  LogicalOperator8/1 -> Switch2/2, RSA_DetectIncrease3/1
  Constant5/1 -> Switch2/1
  LogicalOperator4/1 -> Switch3/2
  Switch2/1 -> Switch3/3
  Add/1 -> Switch3/1
  Constant6/1 -> Add/2
  [EV_CAN_PRESENCE_STARTED] -> LogicalOperator9/1
  [FRAME_INC] -> RSA_DetectChange4/1
  RSA_DetectChange4/1 -> LogicalOperator9/3
  [FRAME_RECEIVED] -> LogicalOperator9/2
  LogicalOperator9/1 -> TIME_OUT_EVENT_AT_INIT2/1
  [FRAME_RECEIVED] -> LogicalOperator12/1
  LogicalOperator12/1 -> LogicalOperator11/3
  TIME_OUT_EVENT_AT_INIT2/1 -> LogicalOperator11/2
  RelationalOperator4/1 -> LogicalOperator13/1
  [FRAME_INC] -> RelationalOperator4/1
  Constant7/1 -> RelationalOperator4/2
  LogicalOperator11/1 -> RSA_DetectIncrease2/1
  RSA_DetectIncrease2/1 -> FRAME_ABSENT/1
  RSA_DetectIncrease3/1 -> FRAME_RECEIVED/1, [FRAME_RECEIVED]
  RSA_DetectChange2/1 -> LogicalOperator1/3
  [EV_CAN_PRESENCE_STARTED] -> LogicalOperator1/1
  Constant3/1 -> TIME_OUT_EVENT_AT_INIT1/2
  Constant8/1 -> TIME_OUT_EVENT_AT_INIT2/2

== system library_BCM/MIL Full Matlab/MUX_SEND_FRAME ==
  CAN_V_EMISSION_ON : Inport  OutDataTypeStr=boolean
      settings: AttributesFormatString=Type : %<OutDataTypeStr>
  EVENT_DATA : Inport  Port=2  OutDataTypeStr=boolean
      settings: AttributesFormatString=Type : %<OutDataTypeStr>
  AND : Logic  AllPortsSameDT=off  OutDataTypeStr=boolean
  Add : Sum  RndMeth=Zero
  Constant1 : Constant  Value=MAX_PARAMETER  OutDataTypeStr=uint8
  Constant10 : Constant  OutDataTypeStr=uint8
  Constant6 : Constant  Value=FRAME_PERIOD  OutDataTypeStr=uint32
  Constant9 : Constant  Value=0  OutDataTypeStr=uint8
  LogicalOperator : Logic  Operator=OR  OutDataTypeStr=boolean
  RelationalOperator2 : RelationalOperator  Operator===  OutDataTypeStr=boolean  InputSameDT=on
  Switch1 : Switch  Criteria=u2 ~= 0  RndMeth=Zero  InputSameDT=on
      settings: AttributesFormatString=Criteria=%<Criteria>
  Switch3 : Switch  Criteria=u2 ~= 0  RndMeth=Zero  InputSameDT=on
      settings: AttributesFormatString=Criteria=%<Criteria>
  TIME_OUT_EVENT_AT_INIT : library_BCM/MIL Full Matlab/TIME_OUT_EVENT_AT_INIT  InitialConditions=true
  UnitDelay1 : UnitDelay  InitialCondition=false  SampleTime=-1
      settings: AttributesFormatString=IC = %<X0>
  FRAME_SEND : Outport  OutDataTypeStr=uint8
      settings: AttributesFormatString=Type : %<OutDataTypeStr>\nInit :%<InitialOutput>
  wires:
  Constant6/1 -> TIME_OUT_EVENT_AT_INIT/2
  TIME_OUT_EVENT_AT_INIT/1 -> LogicalOperator/1, TIME_OUT_EVENT_AT_INIT/1
  Switch1/1 -> Switch3/1
  Switch3/1 -> FRAME_SEND/1, UnitDelay1/1
  [FRAME_SEND] -> Switch3/3
  Add/1 -> Switch1/3
  Constant10/1 -> Add/1
  [FRAME_SEND] -> Add/2, RelationalOperator2/2
  Constant9/1 -> Switch1/1
  EVENT_DATA/1 -> LogicalOperator/2
  Constant1/1 -> RelationalOperator2/1
  RelationalOperator2/1 -> Switch1/2
  UnitDelay1/1 -> [FRAME_SEND]
  CAN_V_EMISSION_ON/1 -> AND/2
  AND/1 -> Switch3/2
  LogicalOperator/1 -> AND/1

== system library_BCM/MIL Full Matlab/NOT_MONITORED_FRAME_MANAGEMENT ==
  FRAME_REC : Inport  OutDataTypeStr=uint32
      settings: AttributesFormatString=Type : %<OutDataTypeStr>
  Constant11 : Constant  Value=65536  OutDataTypeStr=uint32
  Constant2 : Constant  Value=CycleTime  OutDataTypeStr=Inherit: Inherit via back propagation
  LogicalOperator1 : Logic  Operator=OR  OutDataTypeStr=boolean
  LogicalOperator10 : Logic  OutDataTypeStr=boolean
  RSA_DetectChange3 : Renault_Library/Complex blocks/Logic & Bit Operations/RSA_DetectChange  Tag=[LIB]  vinit=65535
      settings: AttributesFormatString=%<MaskType> : Ver : 01.02\nInitial condition: %<vinit>
  RelationalOperator7 : RelationalOperator  OutDataTypeStr=boolean  InputSameDT=on
  TIME_OUT_EVENT_AT_INIT : library_BCM/MIL Full Matlab/TIME_OUT_EVENT_AT_INIT  InitialConditions=true
  FRAME_RECEIVED : Outport  OutDataTypeStr=boolean
      settings: AttributesFormatString=Type : %<OutDataTypeStr>\nInit :%<InitialOutput>
  wires:
  FRAME_REC/1 -> RSA_DetectChange3/1, RelationalOperator7/1
  Constant11/1 -> RelationalOperator7/2
  Constant2/1 -> TIME_OUT_EVENT_AT_INIT/2
  TIME_OUT_EVENT_AT_INIT/1 -> LogicalOperator10/2
  RelationalOperator7/1 -> LogicalOperator10/1
  RSA_DetectChange3/1 -> LogicalOperator1/1
  LogicalOperator10/1 -> LogicalOperator1/2
  LogicalOperator1/1 -> FRAME_RECEIVED/1, TIME_OUT_EVENT_AT_INIT/1

== system library_BCM/MIL Full Matlab/Scheduling ==
  Trigger : TriggerPort  TriggerType=function-call
  Enabled Subsystem : Subsystem  TreatAsAtomicUnit=on
  Lib_Trigger : Subsystem
  Task_XXms : Outport
  wires:
  Enabled Subsystem/1(Out1) -> Task_XXms/1
  Lib_Trigger/1(Out1) -> Enabled Subsystem/Trigger

== system library_BCM/MIL Full Matlab/Scheduling0 ==
  Trigger : TriggerPort  TriggerType=function-call
  Enabled Subsystem : Subsystem  TreatAsAtomicUnit=on
  Lib_Trigger : Subsystem
  Task_XXms : Outport
  wires:
  Lib_Trigger/1(Out1) -> Enabled Subsystem/Enable
  Enabled Subsystem/1(Out1) -> Task_XXms/1

== system library_BCM/MIL Full Matlab/TIME_OUT_EVENT_AT_INIT ==
  In : Inport  OutDataTypeStr=boolean
  dly : Inport  Port=2
  Constant1 : Constant  OutDataTypeStr=Inherit: Inherit via back propagation  SampleTime=-1
  Constant4 : Constant  Value=Ps  SampleTime=-1
  Constant9 : Constant  Value=INIVAL  SampleTime=-1
  DataTypeConversion : DataTypeConversion  OutDataTypeStr=uint32  RndMeth=Zero
  LogicalOperator1 : Logic  Operator=NOT  OutDataTypeStr=boolean
  MinMax : MinMax  Tag=AM,Std,Inputs,1;CMP,Function,Inputs;  Inputs=2  OutDataTypeStr=Inherit: Inherit via back propagation  RndMeth=Zero  SaturateOnIntegerOverflow=on  InputSameDT=on
  MinMax1 : MinMax  Tag=AM,Std,Inputs,1;CMP,Function,Inputs;  Function=max  Inputs=2  OutDataTypeStr=Inherit: Inherit via back propagation  RndMeth=Zero  SaturateOnIntegerOverflow=on  InputSameDT=on
  RSA_DetectDecrease : Renault_Library/Complex blocks/Logic & Bit Operations/RSA_DetectDecrease  Tag=[LIB]  vinit=false
      settings: AttributesFormatString=%<MaskType> : Ver : 01.02\nInitial condition: %<vinit>
  RelationalOperator1 : RelationalOperator  Tag=AM,Std,2,1;CMP,Operator;  Operator===  OutDataTypeStr=boolean  InputSameDT=on
  Sum1 : Sum  OutDataTypeStr=Inherit: Inherit via back propagation  RndMeth=Zero  SaturateOnIntegerOverflow=on  InputSameDT=on
  Sum2 : Sum  Inputs=+-  OutDataTypeStr=Inherit: Inherit via back propagation  RndMeth=Zero  SaturateOnIntegerOverflow=on  InputSameDT=on
  Sum3 : Sum  Inputs=+-  OutDataTypeStr=Inherit: Inherit via back propagation  RndMeth=Zero  SaturateOnIntegerOverflow=on  InputSameDT=on
  Switch1 : Switch  Criteria=u2 ~= 0  RndMeth=Zero  SaturateOnIntegerOverflow=on  InputSameDT=on
      settings: AttributesFormatString=Criteria=%<Criteria>
  UnitDelay : UnitDelay  InitialCondition=InitialConditions  SampleTime=-1
      settings: AttributesFormatString=IC = %<X0>
  UnitDelay1 : UnitDelay  InitialCondition=UDVAL  SampleTime=-1
      settings: AttributesFormatString=IC = %<X0>
  Out : Outport
  wires:
  RSA_DetectDecrease/1 -> UnitDelay/1
  DataTypeConversion/1 -> Sum2/1, MinMax/1
  Constant4/1 -> Sum1/1
  Switch1/1 -> UnitDelay1/1, Sum2/2
  UnitDelay1/1 -> Sum1/2
  Sum1/1 -> Switch1/3
  Constant9/1 -> Switch1/1, [Nsx_Zero]
  In/1 -> Switch1/2
  MinMax/1 -> MinMax1/1
  Sum2/1 -> MinMax/2
  [Nsx_Zero] -> MinMax1/2, RelationalOperator1/2
  MinMax1/1 -> RelationalOperator1/1
  RelationalOperator1/1 -> LogicalOperator1/1
  LogicalOperator1/1 -> RSA_DetectDecrease/1
  UnitDelay/1 -> Out/1
  dly/1 -> Sum3/1
  Sum3/1 -> DataTypeConversion/1
  Constant1/1 -> Sum3/2

== system library_BCM/ModelInfo/EmptySubsystem ==

== system library_BCM/Modeling/Conv_BoolToEvent ==
  Input : Inport  OutDataTypeStr=boolean
  DataTypeConversion : DataTypeConversion  OutDataTypeStr=uint8  RndMeth=Zero
      settings: AttributesFormatString=Saturation:%<SaturateOnIntegerOverflow>
  DataTypeConversion1 : DataTypeConversion  OutDataTypeStr=Enum: TYP_EVENT  RndMeth=Zero
      settings: AttributesFormatString=Saturation:%<SaturateOnIntegerOverflow>
  RSA_DetectChange_v01_04 : Renault_Library/Complex blocks/Logic & Bit Operations/RSA_DetectChange_v01_04  Tag=[LIB]  chkini=on  vinit=false
      settings: AttributesFormatString=%<MaskType> : Ver : 01.04\nCompare the Input with Initial Value = %<chkini>\nInitial Value : = %<vinit>
  Output : Outport  OutDataTypeStr=Enum: TYP_EVENT
      settings: AttributesFormatString=Type : %<OutDataTypeStr>\nInit :%<InitialOutput>
  wires:
  Input/1 -> RSA_DetectChange_v01_04/1
  RSA_DetectChange_v01_04/1 -> DataTypeConversion/1
  DataTypeConversion1/1 -> Output/1
  DataTypeConversion/1 -> DataTypeConversion1/1

== system library_BCM/Modeling/Conv_BoolToEvent_RisingEdge ==
  Input : Inport  OutDataTypeStr=boolean
  DataTypeConversion : DataTypeConversion  OutDataTypeStr=uint8  RndMeth=Zero
      settings: AttributesFormatString=Saturation:%<SaturateOnIntegerOverflow>
  DataTypeConversion1 : DataTypeConversion  OutDataTypeStr=Enum: TYP_EVENT  RndMeth=Zero
      settings: AttributesFormatString=Saturation:%<SaturateOnIntegerOverflow>
  RSA_DetectIncrease_v01_04 : Renault_Library/Complex blocks/Logic & Bit Operations/RSA_DetectIncrease_v01_04  Tag=[LIB]  chkini=off  vinit=false
      settings: AttributesFormatString=%<MaskType> : Ver : 01.04\nCompare the Input with Initial Value = %<chkini>\nInitial Value : = %<vinit>
  Output : Outport  OutDataTypeStr=Enum: TYP_EVENT
      settings: AttributesFormatString=Type : %<OutDataTypeStr>\nInit :%<InitialOutput>
  wires:
  Input/1 -> RSA_DetectIncrease_v01_04/1
  RSA_DetectIncrease_v01_04/1 -> DataTypeConversion/1
  DataTypeConversion1/1 -> Output/1
  DataTypeConversion/1 -> DataTypeConversion1/1

== system library_BCM/Modeling/Conv_EventToBool ==
  Input : Inport  OutDataTypeStr=Enum: TYP_EVENT
      settings: AttributesFormatString=Type : %<OutDataTypeStr>
  DataTypeConversion : DataTypeConversion  OutDataTypeStr=boolean  RndMeth=Zero
      settings: AttributesFormatString=Saturation:%<SaturateOnIntegerOverflow>
  RSA_DetectIncrease_v01_04 : Renault_Library/Complex blocks/Logic & Bit Operations/RSA_DetectIncrease_v01_04  Tag=[LIB]  chkini=on  vinit=false
      settings: AttributesFormatString=%<MaskType> : Ver : 01.04\nCompare the Input with Initial Value = %<chkini>\nInitial Value : = %<vinit>
  Output : Outport  OutDataTypeStr=boolean
      settings: AttributesFormatString=Type : %<OutDataTypeStr>\nInit :%<InitialOutput>
  wires:
  Input/1 -> DataTypeConversion/1
  RSA_DetectIncrease_v01_04/1 -> Output/1
  DataTypeConversion/1 -> RSA_DetectIncrease_v01_04/1

== system library_BCM/Modeling/MPU_BOOLEAN_EXAMPLE ==
  Constant22 : Constant  Value=true  OutDataTypeStr=boolean  SampleTime=-1
  Constant23 : Constant  Value=false  OutDataTypeStr=boolean  SampleTime=-1
  Constant24 : Constant  Value=TYP_MPU_STATUS.MPU_STATUS_DEACTIVATED  OutDataTypeStr=Enum: TYP_MPU_STATUS  SampleTime=-1
  Constant25 : Constant  Value=TYP_MPU_STATUS.MPU_STATUS_ACTIVATED  OutDataTypeStr=Enum: TYP_MPU_STATUS  SampleTime=-1
  Constant26 : Constant  Value=TYP_MPU_REQUEST.MPU_ACTIVATION_REQUEST  OutDataTypeStr=Enum: TYP_MPU_REQUEST  SampleTime=-1
  Constant27 : Constant  Value=TYP_MPU_REQUEST.MPU_RESET_REQUEST  OutDataTypeStr=Enum: TYP_MPU_REQUEST  SampleTime=-1
  Constant28 : Constant  Value=TYP_MPU_REQUEST.MPU_DEACTIVATION_REQUEST  OutDataTypeStr=Enum: TYP_MPU_REQUEST  SampleTime=-1
  Constant29 : Constant  Value=TYP_MPU_REQUEST.MPU_NO_REQUEST  OutDataTypeStr=Enum: TYP_MPU_REQUEST  SampleTime=-1
  Display2 : Display
  EEPROM2 : library_BCM/Validation/EEPROM
  MPU_BOOLEAN : Subsystem
  ManualSwitch16 : ManualSwitch
  ManualSwitch{17..20} (4 alike) : ManualSwitch  CurrentSetting=0
  Scope2 : Scope  NumInputPorts=4
      settings: YMin=-5~-5~-5~-5  YMax=5~5~5~5  SaveName=ScopeData2
  UnitDelay2 : UnitDelay  InitialCondition=TYP_MPU_STATUS.MPU_STATUS_DEACTIVATED  SampleTime=-1
      settings: AttributesFormatString=Initial value : %<X0>
  wires:
  ManualSwitch20/1 -> EEPROM2/1
  ManualSwitch16/1 -> Scope2/3, MPU_BOOLEAN/2(CONFIG_CF)
  MPU_BOOLEAN/1(CUSTOMER_STATUS_S_OUT) -> Scope2/1, UnitDelay2/1, Display2/1
  EEPROM2/1 -> Scope2/4, MPU_BOOLEAN/1(CUSTOMER_STATUS_S)
  Constant22/1 -> ManualSwitch16/1
  Constant23/1 -> ManualSwitch16/2
  Constant28/1 -> ManualSwitch17/1
  Constant26/1 -> ManualSwitch18/1
  Constant29/1 -> ManualSwitch19/2
  Constant27/1 -> ManualSwitch19/1
  Constant25/1 -> ManualSwitch20/1
  Constant24/1 -> ManualSwitch20/2
  UnitDelay2/1 -> EEPROM2/2
  ManualSwitch19/1 -> ManualSwitch17/2
  ManualSwitch17/1 -> ManualSwitch18/2
  ManualSwitch18/1 -> Scope2/2, MPU_BOOLEAN/3(CUSTOMER_REQUEST)

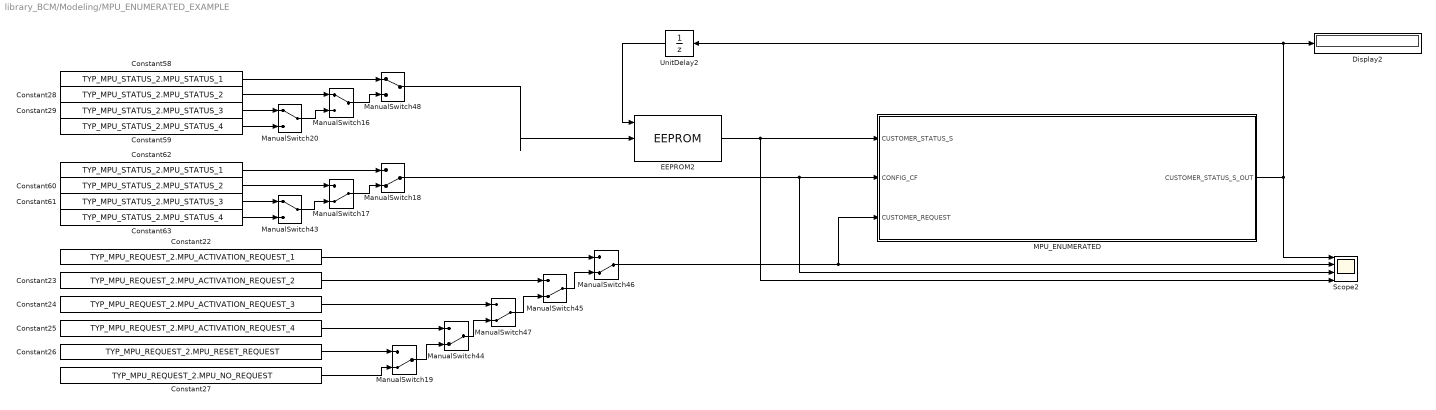
== system library_BCM/Modeling/MPU_ENUMERATED_EXAMPLE ==
  Constant22 : Constant  Value=TYP_MPU_REQUEST_2.MPU_ACTIVATION_REQUEST_1  OutDataTypeStr=Enum: TYP_MPU_REQUEST_2  SampleTime=-1
  Constant23 : Constant  Value=TYP_MPU_REQUEST_2.MPU_ACTIVATION_REQUEST_2  OutDataTypeStr=Enum: TYP_MPU_REQUEST_2  SampleTime=-1
  Constant24 : Constant  Value=TYP_MPU_REQUEST_2.MPU_ACTIVATION_REQUEST_3  OutDataTypeStr=Enum: TYP_MPU_REQUEST_2  SampleTime=-1
  Constant25 : Constant  Value=TYP_MPU_REQUEST_2.MPU_ACTIVATION_REQUEST_4  OutDataTypeStr=Enum: TYP_MPU_REQUEST_2  SampleTime=-1
  Constant26 : Constant  Value=TYP_MPU_REQUEST_2.MPU_RESET_REQUEST  OutDataTypeStr=Enum: TYP_MPU_REQUEST_2  SampleTime=-1
  Constant27 : Constant  Value=TYP_MPU_REQUEST_2.MPU_NO_REQUEST  OutDataTypeStr=Enum: TYP_MPU_REQUEST_2  SampleTime=-1
  Constant28 : Constant  Value=TYP_MPU_STATUS_2.MPU_STATUS_2  OutDataTypeStr=Enum: TYP_MPU_STATUS_2  SampleTime=-1
  Constant29 : Constant  Value=TYP_MPU_STATUS_2.MPU_STATUS_3  OutDataTypeStr=Enum: TYP_MPU_STATUS_2  SampleTime=-1
  Constant58 : Constant  Value=TYP_MPU_STATUS_2.MPU_STATUS_1  OutDataTypeStr=Enum: TYP_MPU_STATUS_2  SampleTime=-1
  Constant59 : Constant  Value=TYP_MPU_STATUS_2.MPU_STATUS_4  OutDataTypeStr=Enum: TYP_MPU_STATUS_2  SampleTime=-1
  Constant60 : Constant  Value=TYP_MPU_STATUS_2.MPU_STATUS_2  OutDataTypeStr=Enum: TYP_MPU_STATUS_2  SampleTime=-1
  Constant61 : Constant  Value=TYP_MPU_STATUS_2.MPU_STATUS_3  OutDataTypeStr=Enum: TYP_MPU_STATUS_2  SampleTime=-1
  Constant62 : Constant  Value=TYP_MPU_STATUS_2.MPU_STATUS_1  OutDataTypeStr=Enum: TYP_MPU_STATUS_2  SampleTime=-1
  Constant63 : Constant  Value=TYP_MPU_STATUS_2.MPU_STATUS_4  OutDataTypeStr=Enum: TYP_MPU_STATUS_2  SampleTime=-1
  Display2 : Display
  EEPROM2 : library_BCM/Validation/EEPROM
  MPU_ENUMERATED : Subsystem
  ManualSwitch{16,20,43,48} (4 alike) : ManualSwitch
  ManualSwitch{17..19,44..47} (7 alike) : ManualSwitch  CurrentSetting=0
  Scope2 : Scope  NumInputPorts=4
      settings: YMin=-5~-5~-5~-5  YMax=5~5~5~5  SaveName=ScopeData5
  UnitDelay2 : UnitDelay  InitialCondition=TYP_MPU_STATUS_2.MPU_STATUS_1  SampleTime=-1
      settings: AttributesFormatString=Initial value : %<X0>
  wires:
  UnitDelay2/1 -> EEPROM2/1
  ManualSwitch48/1 -> EEPROM2/2
  ManualSwitch18/1 -> MPU_ENUMERATED/2(CONFIG_CF), Scope2/3
  MPU_ENUMERATED/1(CUSTOMER_STATUS_S_OUT) -> UnitDelay2/1, Display2/1, Scope2/1
  EEPROM2/1 -> MPU_ENUMERATED/1(CUSTOMER_STATUS_S), Scope2/4
  Constant23/1 -> ManualSwitch45/1
  Constant22/1 -> ManualSwitch46/1
  ManualSwitch44/1 -> ManualSwitch47/2
  Constant24/1 -> ManualSwitch47/1
  ManualSwitch47/1 -> ManualSwitch45/2
  ManualSwitch45/1 -> ManualSwitch46/2
  ManualSwitch46/1 -> Scope2/2, MPU_ENUMERATED/3(CUSTOMER_REQUEST)
  Constant58/1 -> ManualSwitch48/1
  Constant28/1 -> ManualSwitch16/1
  ManualSwitch16/1 -> ManualSwitch48/2
  ManualSwitch17/1 -> ManualSwitch18/2
  Constant25/1 -> ManualSwitch44/1
  Constant26/1 -> ManualSwitch19/1
  Constant27/1 -> ManualSwitch19/2
  ManualSwitch19/1 -> ManualSwitch44/2
  Constant29/1 -> ManualSwitch20/1
  Constant59/1 -> ManualSwitch20/2
  ManualSwitch20/1 -> ManualSwitch16/2
  ManualSwitch43/1 -> ManualSwitch17/2
  Constant61/1 -> ManualSwitch43/1
  Constant63/1 -> ManualSwitch43/2
  Constant62/1 -> ManualSwitch18/1
  Constant60/1 -> ManualSwitch17/1
